simulink model "test_EN12977_StorageType1_Strat"  (R2018b)
settings: Solver=ode45  StartTime=time(1)  StopTime=time(end)  MaxStep=time(2)-time(1)  RelTol=1e-3  EnableMultiTasking=on
undefined symbols (not defined in the file or in its folder): Tstg
libraries: carnot x12
settings Model: Creator=drhf  LastModifiedBy=P41573
settings DataIOCC: LimitDataPoints=on  SaveFormat=Array  SaveOutput=off  SaveTime=off
settings OptimizationCC: ExpressionDepthLimit=2147483647  LifeSpan=inf
settings DebuggingCC: UnderspecifiedInitializationDetection=Classic  MergeDetectMultiDrivingBlocksExec=none  SolverPrmCheckMsg=warning  StateNameClashWarn=warning  SFUnexpectedBacktrackingDiag=warning  SFNoUnconditionalDefaultTransitionDiag=warning  SFExecutionAtInitializationDiag=none
settings HardwareCC: ProdBitPerPointer=32  ProdBitPerSizeT=32  ProdBitPerPtrDiffT=32  ProdLargestAtomicFloat=None  ProdIntDivRoundTo=Undefined  ProdEndianess=Unspecified  ProdWordSize=32  ProdHWDeviceType=32-bit Generic
settings ModelReferenceCC: PropagateSignalLabelsOutOfModel=off
settings SFSimCC: SimUseLocalCustomCode=off
settings RTWCC: RTWUseLocalCustomCode=off
settings CodeAppCC: StateflowObjectComments=on
settings GRTTargetCC: TargetLangStandard=C89/C90 (ANSI)  GeneratePreprocessorConditionals=Disable all  CombineOutputUpdateFcns=off  GRTInterface=on
settings ConfigComp: CovMetricSettings=dw  CovHtmlReporting=on  CovSaveCumulativeToWorkspaceVar=on  CovSaveSingleToWorkspaceVar=on  CovExternalEMLEnable=off

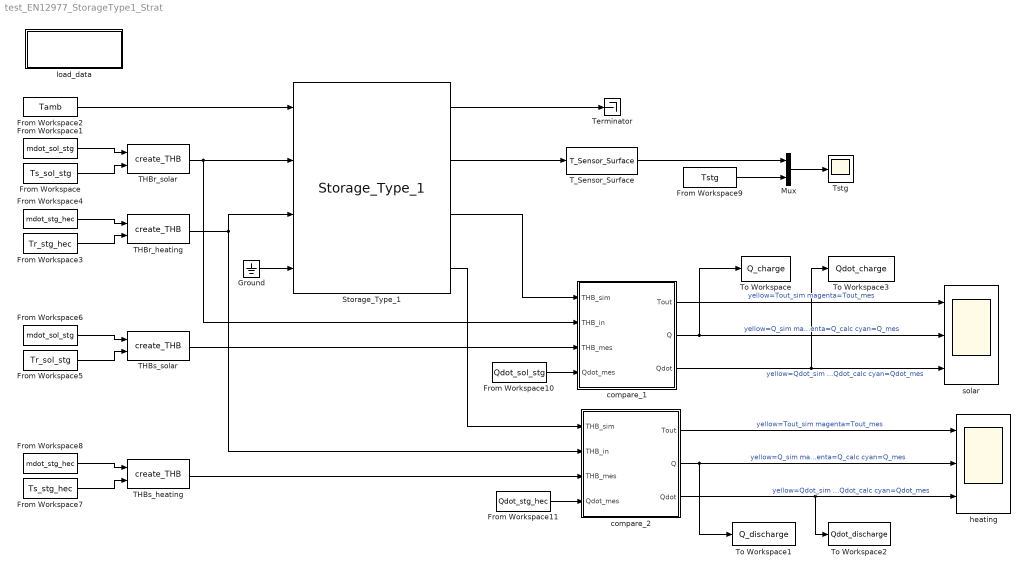
== system test_EN12977_StorageType1_Strat ==
  From Workspace : FromWorkspace  VariableName=Ts_sol_stg  SampleTime=0
  From Workspace1 : FromWorkspace  VariableName=mdot_sol_stg  SampleTime=0
  From Workspace10 : FromWorkspace  VariableName=Qdot_sol_stg  SampleTime=0
  From Workspace11 : FromWorkspace  VariableName=Qdot_stg_hec  SampleTime=0
  From Workspace2 : FromWorkspace  VariableName=Tamb  SampleTime=0
  From Workspace3 : FromWorkspace  VariableName=Tr_stg_hec  SampleTime=0
  From Workspace4 : FromWorkspace  VariableName=mdot_stg_hec  SampleTime=0
  From Workspace5 : FromWorkspace  VariableName=Tr_sol_stg  SampleTime=0
  From Workspace6 : FromWorkspace  VariableName=mdot_sol_stg  SampleTime=0
  From Workspace7 : FromWorkspace  VariableName=Ts_stg_hec  SampleTime=0
  From Workspace8 : FromWorkspace  VariableName=mdot_stg_hec  SampleTime=0
  From Workspace9 : FromWorkspace  VariableName=Tstg  SampleTime=0
  Ground : Ground
  Mux : Mux  Inputs=2
  Storage_Type_1 : carnot/Storage/Thermal/Storage_Type_1  t0=interp1(1:10, Tstg(1, 2:end), 10:-9/99:1)  hgt=0.9972  stgtype=1  tini=[20.2837 20.2844818181818 20.2852636363636 20.2860454545455 20.2868272727273 20.2876090909091 20.2883909090909 20.2891727272727 20.2899545454545 20.2907363636364 20.2915181818182 20.2923 20.2901090909091 20.2879181818182 20.2857272727273 20.2835363636364 20.2813454545455 20.2791545454545 20.2769636363636 20.2747727272727 20.2725818181818 20.2703909090909 20.2682 20.2781181818182 20.2880363636364 20.2979545454545 20.3078727272727 20.3177909090909 20.3277090909091 20.3376272727273 20.3475454545455 20.3574636363636 20.3673818181818 20.3773 20.3429545454545 20.3086090909091 20.2742636363636 20.2399181818182 20.2055727272727 20.1712272727273 20.1368818181818 20.1025363636364 20.0681909090909 20.0338454545455 19.9995 20.0215272727273 20.0435545454545 20.0655818181818 20.0876090909091 20.1096363636364 20.1316636363636 20.1536909090909 20.1757181818182 20.1977454545455 20.2197727272727 20.2418 20.2546727272727 20.2675454545455 20.2804181818182 20.2932909090909 20.3061636363636 20.3190363636364 20.3319090909091 20.3447818181818 20.3576545454545 20.3705272727273 20.3834 20.3654545454545 20.3475090909091 20.3295636363636 20.3116181818182 20.2936727272727 20.2757272727273 20.2577818181818 20.2398363636364 20.2218909090909 20.2039454545455 20.186 20.1829090909091 20.1798181818182 20.1767272727273 20.1736363636364 20.1705454545455 20.1674545454545 20.1643636363636 20.1612727272727 20.1581818181818 20.1550909090909 20.152 20.1464818181818 20.1409636363636 20.1354454545455 20.1299272727273 20.1244090909091 20.1188909090909 20.1133727272727 20.1078545454545 20.1023363636364 20.0968181818182 20.0913]  mpts=[3 8 13 18 23 28 33 38 43 48 53 58 63 68 73 78 83 88 93 98]  PathName='current'  FileName='Stg_verification_param.mat'  userPath=off  userParam=off  uwall=1.4  ubot=1.4  utop=1.4  axcond=1.2  volume=0.22  dia=0.53  standing=standing cylinder  nodes=100  mpoints=20  Tsensor=0.5  pipe1inlet=0.62  pipe1outlet=0  pipe1dia=0.03  pipe2inlet=0.1  pipe2outlet=1  pipe2dia=0.03  heater1start=0.6  heater1end=0.65
      settings: SourceProductName=Carnot
  THBr_heating : carnot/Source/Simple/create_THB  p=1e5  fluid=Water  mix=0  mix2=0  mix3=0  dia=0.02  hgt=0  mID=No Pressure Drop
      settings: SourceProductName=Carnot
  THBr_solar : carnot/Source/Simple/create_THB  p=1e5  fluid=Water  mix=0  mix2=0  mix3=0  dia=0.02  hgt=0  mID=No Pressure Drop
      settings: SourceProductName=Carnot
  THBs_heating : carnot/Source/Simple/create_THB  p=1e5  fluid=Water  mix=0  mix2=0  mix3=0  dia=0.02  hgt=0  mID=No Pressure Drop
      settings: SourceProductName=Carnot
  THBs_solar : carnot/Source/Simple/create_THB  p=1e5  fluid=Water  mix=0  mix2=0  mix3=0  dia=0.02  hgt=0  mID=No Pressure Drop
      settings: SourceProductName=Carnot
  T_Sensor_Surface : carnot/Control/T_Sensor_Surface  pos=[0.8830 0.7980 0.7130 0.6280 0.5430 0.4570 0.3720 0.2870 0.2020 0.1170]  tdel=1  t0=Tstg(1, 2:11)
      settings: SourceProductName=Carnot
  Terminator : Terminator
  To Workspace : ToWorkspace  VariableName=Q_charge  SampleTime=-1
      settings: MaxDataPoints=1
  To Workspace1 : ToWorkspace  VariableName=Q_discharge  SampleTime=-1
      settings: MaxDataPoints=1
  To Workspace2 : ToWorkspace  VariableName=Qdot_discharge  SampleTime=180
  To Workspace3 : ToWorkspace  VariableName=Qdot_charge  SampleTime=180
  Tstg : Scope
  compare_1 : Subsystem
  compare_2 : Subsystem
  heating : Scope  NumInputPorts=3
  load_data : Subsystem
      settings: OpenFcn=|
      | [filename, pathname, filterindex] = ...
      |    uigetfile( {  'data*.mat', ...
      |    'validation files (data*.mat)'; ...
      |    '*.mat','MAT-files (*.mat)'; ...
      |    '*.*',  'All Files (*.*)'},  'Pick a data file');
      | 
      | if (filterindex > 0)
      |    load(filename)
      | end
      mask Display: disp('double click \nto load data')
  solar : Scope  NumInputPorts=3
  wires:
  Storage_Type_1/1 -> Terminator/1
  Storage_Type_1/2 -> T_Sensor_Surface/1
  From Workspace2/1 -> Storage_Type_1/1
  THBr_solar/1 -> Storage_Type_1/2, compare_1/2(THB_in)
  THBr_heating/1 -> Storage_Type_1/3, compare_2/2(THB_in)
  compare_1/1(Tout) -> solar/1  "yellow=Tout_sim magenta=Tout_mes"
  compare_1/2(Q) -> solar/2, To Workspace/1  "yellow=Q_sim magenta=Q_calc cyan=Q_mes"
  Storage_Type_1/3 -> compare_1/1(THB_sim)
  THBs_solar/1 -> compare_1/3(THB_mes)
  compare_2/1(Tout) -> heating/1  "yellow=Tout_sim magenta=Tout_mes"
  compare_2/2(Q) -> heating/2, To Workspace1/1  "yellow=Q_sim magenta=Q_calc cyan=Q_mes"
  THBs_heating/1 -> compare_2/3(THB_mes)
  Storage_Type_1/4 -> compare_2/1(THB_sim)
  Mux/1 -> Tstg/1
  T_Sensor_Surface/1 -> Mux/1
  From Workspace9/1 -> Mux/2
  compare_1/3(Qdot) -> solar/3, To Workspace3/1  "yellow=Qdot_sim magenta=Qdot_calc cyan=Qdot_mes"
  From Workspace10/1 -> compare_1/4(Qdot_mes)
  From Workspace11/1 -> compare_2/4(Qdot_mes)
  compare_2/3(Qdot) -> heating/3, To Workspace2/1  "yellow=Qdot_sim magenta=Qdot_calc cyan=Qdot_mes"
  From Workspace1/1 -> THBr_solar/1
  From Workspace/1 -> THBr_solar/2
  From Workspace4/1 -> THBr_heating/1
  From Workspace3/1 -> THBr_heating/2
  From Workspace6/1 -> THBs_solar/1
  From Workspace5/1 -> THBs_solar/2
  From Workspace8/1 -> THBs_heating/1
  From Workspace7/1 -> THBs_heating/2
  Ground/1 -> Storage_Type_1/4

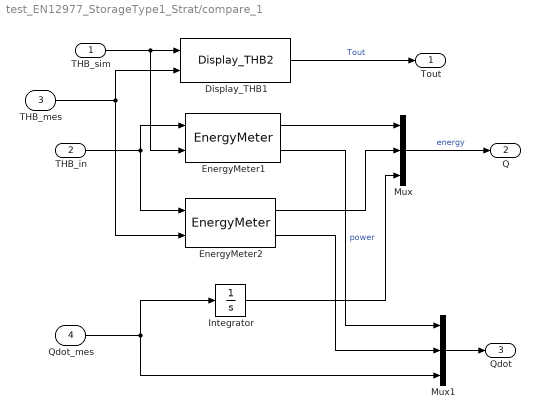
== system test_EN12977_StorageType1_Strat/compare_1 ==
  THB_sim : Inport
  THB_in : Inport  Port=2
  THB_mes : Inport  Port=3
  Qdot_mes : Inport  Port=4
  Display_THB1 : carnot/Outputs/Display_THB2  t=on  m=off  p=off  id=off  mix=off  d=off
      settings: SourceProductName=Carnot
  EnergyMeter1 : carnot/Control/EnergyMeter
      settings: SourceProductName=Carnot
  EnergyMeter2 : carnot/Control/EnergyMeter
      settings: SourceProductName=Carnot
  Integrator : Integrator  UpperSaturationLimit=1  LowerSaturationLimit=0
  Mux : Mux  Inputs=3
  Mux1 : Mux  Inputs=3
  Tout : Outport
  Q : Outport  Port=2
  Qdot : Outport  Port=3
  wires:
  THB_sim/1 -> EnergyMeter1/2, Display_THB1/1
  THB_mes/1 -> EnergyMeter2/2, Display_THB1/2
  EnergyMeter1/1 -> Mux/1
  Display_THB1/1 -> Tout/1  "Tout"
  Mux/1 -> Q/1  "energy"
  Qdot_mes/1 -> Integrator/1, Mux1/3
  EnergyMeter1/2 -> Mux1/1  "power"
  Mux1/1 -> Qdot/1
  THB_in/1 -> EnergyMeter2/1, EnergyMeter1/1
  EnergyMeter2/1 -> Mux/2
  EnergyMeter2/2 -> Mux1/2
  Integrator/1 -> Mux/3

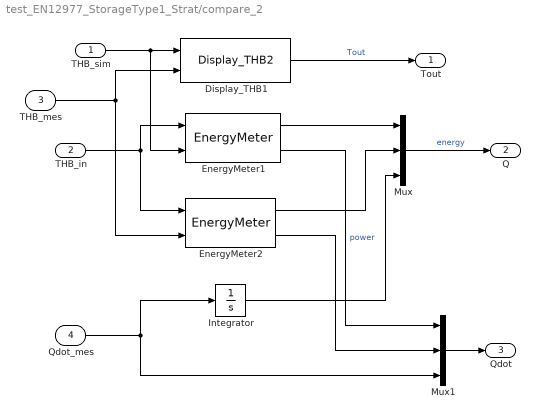
== system test_EN12977_StorageType1_Strat/compare_2 ==
  THB_sim : Inport
  THB_in : Inport  Port=2
  THB_mes : Inport  Port=3
  Qdot_mes : Inport  Port=4
  Display_THB1 : carnot/Outputs/Display_THB2  t=on  m=off  p=off  id=off  mix=off  d=off
      settings: SourceProductName=Carnot
  EnergyMeter1 : carnot/Control/EnergyMeter
      settings: SourceProductName=Carnot
  EnergyMeter2 : carnot/Control/EnergyMeter
      settings: SourceProductName=Carnot
  Integrator : Integrator  UpperSaturationLimit=1  LowerSaturationLimit=0
  Mux : Mux  Inputs=3
  Mux1 : Mux  Inputs=3
  Tout : Outport
  Q : Outport  Port=2
  Qdot : Outport  Port=3
  wires:
  Integrator/1 -> Mux/3
  EnergyMeter2/2 -> Mux1/2
  EnergyMeter2/1 -> Mux/2
  THB_in/1 -> EnergyMeter1/1, EnergyMeter2/1
  Mux1/1 -> Qdot/1
  EnergyMeter1/2 -> Mux1/1  "power"
  Qdot_mes/1 -> Mux1/3, Integrator/1
  Mux/1 -> Q/1  "energy"
  Display_THB1/1 -> Tout/1  "Tout"
  EnergyMeter1/1 -> Mux/1
  THB_mes/1 -> Display_THB1/2, EnergyMeter2/2
  THB_sim/1 -> Display_THB1/1, EnergyMeter1/2

== system test_EN12977_StorageType1_Strat/load_data ==
